simulink model "MPC_Validation_2"  (R2020a)
settings: Solver=FixedStepAuto  StartTime=0.0  StopTime=tsim  FixedStep=baseRate  RelTol=1e-3  EnableMultiTasking=on
values from neighbouring files (symbols this model uses):
  Ad = -C(7:12,4:9)    [theFastMPCSolver3.m]
  ALGORITHM = 5    [Run_Initializer.m]    (also in main.m = 7)
  baseRate = 0.05    [Run_Initializer.m]
  con0 = [n*N, 2*N, N, N, N]    [Run_Initializer.m]    (also in main.m)
  drop_states_ARM = [ pi/2, pi/2, 0]    [Run_Initializer.m]
  drop_states_BLACK = rand([1,3])/10+init_states_BLACK    [Run_Initializer.m]
  drop_states_BLUE = rand([1,3])/10+init_states_BLUE    [Run_Initializer.m]
  drop_states_RED = rand([1,3])/10+init_states_RED    [Run_Initializer.m]
  F_Black_X_nominal = 0.2196    [Run_Initializer.m]
  F_Black_Y_nominal = 0.2825    [Run_Initializer.m]
  F_Blue_X_nominal = 0.2196    [Run_Initializer.m]
  F_Blue_Y_nominal = 0.2825    [Run_Initializer.m]
  F_red_X_nominal = 0.2196    [Run_Initializer.m]
  F_red_Y_nominal = 0.2825    [Run_Initializer.m]
  F_thrusters_BLACK = [F_Black_X_nominal; F_Black_X_nominal;                             F_Black_Y_nominal; F_Black_Y_nominal; F_Black_X_nominal;                              F_Black_X_nominal; F_Black_Y_nominal; F_Black_Y_nominal]    [Run_Initializer.m]
  F_thrusters_BLUE = [F_Blue_X_nominal; F_Blue_X_nominal;                             F_Blue_Y_nominal; F_Blue_Y_nominal; F_Blue_X_nominal;                              F_Blue_X_nominal; F_Blue_Y_nominal; F_Blue_Y_nominal]    [Run_Initializer.m]
  F_thrusters_RED = [F_red_X_nominal; F_red_X_nominal;                             F_red_Y_nominal; F_red_Y_nominal; F_red_X_nominal;                              F_red_X_nominal; F_red_Y_nominal; F_red_Y_nominal]    [Run_Initializer.m]
  gamma = r - (excess + shrink + bracketwidth)    [theChaserSpacecraft.m]    (also in theTargetSpacecraft.m)
  Gamma1 = 0.0025    [Run_Initializer.m]
  Gamma2 = 100    [Run_Initializer.m]
  Gamma3 = 10    [Run_Initializer.m]
  Gamma4 = 0.001    [Run_Initializer.m]
  Gamma5 = 100    [Run_Initializer.m]
  Gamma6 = 0.001    [Run_Initializer.m]
  init_states_BLACK = [ct;thetat0].'    [Run_Initializer.m]
  init_states_BLUE = [pobj1;0].'    [Run_Initializer.m]
  init_states_RED = xi(1:3).'    [Run_Initializer.m]
  Kd_elarm = 0.05    [Run_Initializer.m]
  Kd_sharm = 0.05    [Run_Initializer.m]
  Kd_tb = 0.4    [Run_Initializer.m]
  Kd_tblue = 0.4    [Run_Initializer.m]
  Kd_tr = 0.4    [Run_Initializer.m]
  Kd_wrarm = 0.005    [Run_Initializer.m]
  Kd_xb = 8    [Run_Initializer.m]
  Kd_xblue = 8    [Run_Initializer.m]
  Kd_xr = 8    [Run_Initializer.m]
  Kd_yb = 8    [Run_Initializer.m]
  Kd_yblue = 8    [Run_Initializer.m]
  Kd_yr = 8    [Run_Initializer.m]
  Kp = [0.08 0 0 ... (first row only)    [Run_Initializer.m]
  Kp_elarm = 0.08    [Run_Initializer.m]
  Kp_sharm = 0.15    [Run_Initializer.m]
  Kp_tb = 0.1    [Run_Initializer.m]
  Kp_tblue = 0.1    [Run_Initializer.m]
  Kp_tr = 0.1    [Run_Initializer.m]
  Kp_wrarm = 0.007    [Run_Initializer.m]
  Kp_xb = 2    [Run_Initializer.m]
  Kp_xblue = 2    [Run_Initializer.m]
  Kp_xr = 2    [Run_Initializer.m]
  Kp_yb = 2    [Run_Initializer.m]
  Kp_yblue = 2    [Run_Initializer.m]
  Kp_yr = 2    [Run_Initializer.m]
  Kv = [0.05 0 0 ... (first row only)    [Run_Initializer.m]
  maxiterations = 10    [Run_Initializer.m]    (also in main.m)
  N = 15    [Run_Initializer.m]    (also in main.m; theFastMPCSolver2.m = length(z)/9; theFastMPCSolver3.m = length(z)/9)
  n = size(b,1)    [theFastMPCSolver3.m]
  noise_variance_BLACK = 0    [Run_Initializer.m]
  noise_variance_BLUE = 0    [Run_Initializer.m]
  noise_variance_RED = 0    [Run_Initializer.m]
  Phase0_End = Phase0_Duration    (= 5)    [Run_Initializer.m]
  Phase1_End = Phase0_Duration + Phase1_Duration    (= 10)    [Run_Initializer.m]
  Phase2_End = Phase0_Duration + Phase1_Duration +                                   Phase2_Duration    (= 36)    [Run_Initializer.m]
  Phase3_End = Phase0_Duration + Phase1_Duration +                                   Phase2_Duration + Phase3_Duration    (= 166)    [Run_Initializer.m]
  Phase3_SubPhase1_End = Phase2_End + Phase3_SubPhase1_Duration    (= 40)    [Run_Initializer.m]
  Phase3_SubPhase2_End = Phase2_End + Phase3_SubPhase1_Duration +                                   Phase3_SubPhase2_Duration    (= 42)    [Run_Initializer.m]
  Phase3_SubPhase3_End = Phase2_End + Phase3_SubPhase1_Duration +                                   Phase3_SubPhase2_Duration +                                  Phase3_SubPhase3_Duration    (= 44)    [Run_Initializer.m]
  Phase3_SubPhase4_End = Phase2_End + Phase3_SubPhase1_Duration +                                   Phase3_SubPhase2_Duration +                                  Phase3_SubPhase3_Duration +                                  Phase3_SubPhase4_Duration    [Run_Initializer.m]
  Phase4_End = Phase0_Duration + Phase1_Duration +                                   Phase2_Duration + Phase3_Duration +                                   Phase4_Duration    (= 186)    [Run_Initializer.m]
  Phase5_End = Phase0_Duration + Phase1_Duration +                                   Phase2_Duration + Phase3_Duration +                                   Phase4_Duration + Phase5_Duration    (= 191)    [Run_Initializer.m]
  serverRate = 0.1    [Run_Initializer.m]
  Td = 2    [Run_Initializer.m]    (also in main.m)
  thetat_dot = 0 * d2r    (= 0)    [Run_Initializer.m]    (also in main.m = -2.0 * d2r)
  thruster_dist2CG_BLACK = [83.42;-52.58;55.94;-60.05;54.08;-53.92;77.06;-55.94]    [Run_Initializer.m]
  thruster_dist2CG_BLUE = [73.54;-64.46;81.39;-60.11;64.46;-65.94;54.61;-74.39]    [Run_Initializer.m]
  thruster_dist2CG_RED = [49.92;-78.08;70.46;-63.54;81.08;-50.42;57.44;-75.96]    [Run_Initializer.m]
  tol = 0.00015    [Run_Initializer.m]    (also in main.m)
  Tz_lim_elarm = .1    (= 0.1)    [Run_Initializer.m]
  Tz_lim_sharm = .1    (= 0.1)    [Run_Initializer.m]
  Tz_lim_wrarm = .1    (= 0.1)    [Run_Initializer.m]
  vobj1 = [0.00;0.00]    [Run_Initializer.m]    (also in main.m)
  vtar = [0.0;0.0]    [Run_Initializer.m]    (also in main.m = [-0.008;0.008])
undefined symbols (not defined in the file or in its folder): cdockdeltax, cdockoa, Cmat, DiscIntNeverNeededParam, ecoa, Fmat, H, KOZ_actual, model_param, pdockoa, pdockr, platformSelection, rcone, rdock, simMode, Sj, taumax, thetah, Umat, umax, WhoAmI
libraries: dspstat3 x23, dspsigops x15, embdlinuxlib x10, raspberrypiBasiclib x10, simulink x8, MainLibrary x7, mspfiltlib x3, dsparch4 x3, dspswit3 x2, sensehatlib x1
(part 7 of 14)

== system MPC_Validation_2/IMU Data and Algorithms/Change RED Behavior/Fix Initial Bias/Correct GyroZ ==
  In1 : Inport
  Calculate Running Mean : Subsystem  TreatAsAtomicUnit=on
  Compare To Zero1 : simulink/Logic and Bit Operations/Compare To Zero  relop===  OutDataTypeStr=boolean
  Data Store Read1 : DataStoreRead  DataStoreName=RED_Rz
  Data Store Read3 : DataStoreRead  DataStoreName=RED_IMU_R
  Discrete-Time Integrator1 : DiscreteIntegrator  IntegratorMethod=Integration: Backward Euler  ExternalReset=either  InitialConditionSource=external  SampleTime=-1  ICPrevOutput=DiscIntNeverNeededParam  ICPrevScaledInput=DiscIntNeverNeededParam
  If : If  IfExpression=u1 < 5
  Pass Current Gyro : Subsystem  TreatAsAtomicUnit=on
  RED_Px4 : DataStoreWrite  DataStoreName=RED_IMU_Psi
  Subsystem : Subsystem
  Subtract : Sum  Inputs=+-
  Out1 : Outport
  wires:
  Subtract/1 -> Out1/1
  Subsystem/1(Time) -> If/1
  If/2 -> Pass Current Gyro/Action
  In1/1 -> Calculate Running Mean/1(In1), Pass Current Gyro/1(In1)
  If/1 -> Calculate Running Mean/Action
  Calculate Running Mean/1(Out1) -> Subtract/2
  Discrete-Time Integrator1/1 -> RED_Px4/1
  Compare To Zero1/1 -> Discrete-Time Integrator1/2
  Pass Current Gyro/1(Out1) -> Compare To Zero1/1, Subtract/1
  Data Store Read3/1 -> Discrete-Time Integrator1/1
  Data Store Read1/1 -> Discrete-Time Integrator1/3

== system MPC_Validation_2/IMU Data and Algorithms/Change RED Behavior/Fix Initial Bias (Accel)/Correct AccelX ==
  In1 : Inport
  Calculate Running Mean : Subsystem  TreatAsAtomicUnit=on
  If : If  IfExpression=u1 < 5
  Pass Current Accel : Subsystem  TreatAsAtomicUnit=on
  Subsystem : Subsystem
  Subtract : Sum  Inputs=+-
  Out1 : Outport
  wires:
  Subtract/1 -> Out1/1
  Subsystem/1(Time) -> If/1
  If/2 -> Pass Current Accel/Action
  In1/1 -> Calculate Running Mean/1(In1), Pass Current Accel/1(In1)
  If/1 -> Calculate Running Mean/Action
  Pass Current Accel/1(Out1) -> Subtract/1
  Calculate Running Mean/1(Out1) -> Subtract/2

== system MPC_Validation_2/IMU Data and Algorithms/Change RED Behavior/Fix Initial Bias (Accel)/Correct AccelY ==
  In1 : Inport
  Calculate Running Mean : Subsystem  TreatAsAtomicUnit=on
  If : If  IfExpression=u1 < 5
  Pass Current Accel : Subsystem  TreatAsAtomicUnit=on
  Subsystem : Subsystem
  Subtract : Sum  Inputs=+-
  Out1 : Outport
  wires:
  Subtract/1 -> Out1/1
  Subsystem/1(Time) -> If/1
  If/2 -> Pass Current Accel/Action
  In1/1 -> Calculate Running Mean/1(In1), Pass Current Accel/1(In1)
  If/1 -> Calculate Running Mean/Action
  Pass Current Accel/1(Out1) -> Subtract/1
  Calculate Running Mean/1(Out1) -> Subtract/2

== system MPC_Validation_2/IMU Data and Algorithms/Change RED Behavior/Fix Initial Bias (Accel)/Correct AccelZ ==
  In1 : Inport
  Calculate Running Mean : Subsystem  TreatAsAtomicUnit=on
  If : If  IfExpression=u1 < 5
  Pass Current Accel : Subsystem  TreatAsAtomicUnit=on
  Subsystem : Subsystem
  Subtract : Sum  Inputs=+-
  Out1 : Outport
  wires:
  Subtract/1 -> Out1/1
  Subsystem/1(Time) -> If/1
  If/2 -> Pass Current Accel/Action
  In1/1 -> Calculate Running Mean/1(In1), Pass Current Accel/1(In1)
  If/1 -> Calculate Running Mean/Action
  Pass Current Accel/1(Out1) -> Subtract/1
  Calculate Running Mean/1(Out1) -> Subtract/2

== system MPC_Validation_2/Phase #2: Move to Initial Position/Change BLACK Behavior/Custom Discrete PD (Attitude)/x_dot -> x1 ==
  note: dy/dt ~= (y2-y1)/deltaT
  y(t) : Inport
  Delay1 : Delay  DelayLength=1  InitialConditionSource=Input port
      settings: InputPortMap=u0,p4
  Hold this value : Subsystem  TreatAsAtomicUnit=on
  Sum6 : Sum  Inputs=-+|
  divide by delta T : Gain  Gain=1/serverRate
  "if we went through a \"step\"" : If  IfExpression=u1 ~= 0  ShowElse=off
  dy(t)/dt : Outport  VectorParamsAs1DForOutWhenUnconnected=off
  wires:
  divide by delta T/1 -> dy(t)/dt/1
  Delay1/1 -> Sum6/1
  "if we went through a \"step\""/1 -> Hold this value/Action
  Hold this value/1(Out1) -> divide by delta T/1
  Sum6/1 -> "if we went through a \"step\""/1, Hold this value/1(In1)
  y(t)/1 -> Sum6/2, Delay1/2, Delay1/1

== system MPC_Validation_2/Phase #2: Move to Initial Position/Change BLACK Behavior/Custom Discrete PD (X-Position)/x_dot -> x1 ==
  note: dy/dt ~= (y2-y1)/deltaT
  y(t) : Inport
  Delay1 : Delay  DelayLength=1  InitialConditionSource=Input port
      settings: InputPortMap=u0,p4
  Hold this value : Subsystem  TreatAsAtomicUnit=on
  Sum6 : Sum  Inputs=-+|
  divide by delta T : Gain  Gain=1/serverRate
  "if we went through a \"step\"" : If  IfExpression=u1 ~= 0  ShowElse=off
  dy(t)/dt : Outport  VectorParamsAs1DForOutWhenUnconnected=off
  wires:
  divide by delta T/1 -> dy(t)/dt/1
  Delay1/1 -> Sum6/1
  "if we went through a \"step\""/1 -> Hold this value/Action
  Hold this value/1(Out1) -> divide by delta T/1
  Sum6/1 -> "if we went through a \"step\""/1, Hold this value/1(In1)
  y(t)/1 -> Sum6/2, Delay1/2, Delay1/1

== system MPC_Validation_2/Phase #2: Move to Initial Position/Change BLACK Behavior/Custom Discrete PD (Y-Position)/x_dot -> x1 ==
  note: dy/dt ~= (y2-y1)/deltaT
  y(t) : Inport
  Delay1 : Delay  DelayLength=1  InitialConditionSource=Input port
      settings: InputPortMap=u0,p4
  Hold this value : Subsystem  TreatAsAtomicUnit=on
  Sum6 : Sum  Inputs=-+|
  divide by delta T : Gain  Gain=1/serverRate
  "if we went through a \"step\"" : If  IfExpression=u1 ~= 0  ShowElse=off
  dy(t)/dt : Outport  VectorParamsAs1DForOutWhenUnconnected=off
  wires:
  divide by delta T/1 -> dy(t)/dt/1
  Delay1/1 -> Sum6/1
  "if we went through a \"step\""/1 -> Hold this value/Action
  Hold this value/1(Out1) -> divide by delta T/1
  Sum6/1 -> "if we went through a \"step\""/1, Hold this value/1(In1)
  y(t)/1 -> Sum6/2, Delay1/2, Delay1/1

== system MPC_Validation_2/Phase #2: Move to Initial Position/Change BLUE Behavior/Custom Discrete PD (Attitude)/x_dot -> x1 ==
  note: dy/dt ~= (y2-y1)/deltaT
  y(t) : Inport
  Delay1 : Delay  DelayLength=1  InitialConditionSource=Input port
      settings: InputPortMap=u0,p4
  Hold this value : Subsystem  TreatAsAtomicUnit=on
  Sum6 : Sum  Inputs=-+|
  divide by delta T : Gain  Gain=1/serverRate
  "if we went through a \"step\"" : If  IfExpression=u1 ~= 0  ShowElse=off
  dy(t)/dt : Outport  VectorParamsAs1DForOutWhenUnconnected=off
  wires:
  divide by delta T/1 -> dy(t)/dt/1
  Delay1/1 -> Sum6/1
  "if we went through a \"step\""/1 -> Hold this value/Action
  Hold this value/1(Out1) -> divide by delta T/1
  Sum6/1 -> "if we went through a \"step\""/1, Hold this value/1(In1)
  y(t)/1 -> Sum6/2, Delay1/2, Delay1/1

== system MPC_Validation_2/Phase #2: Move to Initial Position/Change BLUE Behavior/Custom Discrete PD (X-Position)/x_dot -> x1 ==
  note: dy/dt ~= (y2-y1)/deltaT
  y(t) : Inport
  Delay1 : Delay  DelayLength=1  InitialConditionSource=Input port
      settings: InputPortMap=u0,p4
  Hold this value : Subsystem  TreatAsAtomicUnit=on
  Sum6 : Sum  Inputs=-+|
  divide by delta T : Gain  Gain=1/serverRate
  "if we went through a \"step\"" : If  IfExpression=u1 ~= 0  ShowElse=off
  dy(t)/dt : Outport  VectorParamsAs1DForOutWhenUnconnected=off
  wires:
  divide by delta T/1 -> dy(t)/dt/1
  Delay1/1 -> Sum6/1
  "if we went through a \"step\""/1 -> Hold this value/Action
  Hold this value/1(Out1) -> divide by delta T/1
  Sum6/1 -> "if we went through a \"step\""/1, Hold this value/1(In1)
  y(t)/1 -> Sum6/2, Delay1/2, Delay1/1

== system MPC_Validation_2/Phase #2: Move to Initial Position/Change BLUE Behavior/Custom Discrete PD (Y-Position)/x_dot -> x1 ==
  note: dy/dt ~= (y2-y1)/deltaT
  y(t) : Inport
  Delay1 : Delay  DelayLength=1  InitialConditionSource=Input port
      settings: InputPortMap=u0,p4
  Hold this value : Subsystem  TreatAsAtomicUnit=on
  Sum6 : Sum  Inputs=-+|
  divide by delta T : Gain  Gain=1/serverRate
  "if we went through a \"step\"" : If  IfExpression=u1 ~= 0  ShowElse=off
  dy(t)/dt : Outport  VectorParamsAs1DForOutWhenUnconnected=off
  wires:
  divide by delta T/1 -> dy(t)/dt/1
  Delay1/1 -> Sum6/1
  "if we went through a \"step\""/1 -> Hold this value/Action
  Hold this value/1(Out1) -> divide by delta T/1
  Sum6/1 -> "if we went through a \"step\""/1, Hold this value/1(In1)
  y(t)/1 -> Sum6/2, Delay1/2, Delay1/1

== system MPC_Validation_2/Phase #2: Move to Initial Position/Change RED Behavior/Custom Discrete PD (Attitude)/x_dot -> x1 ==
  note: dy/dt ~= (y2-y1)/deltaT
  y(t) : Inport
  Delay1 : Delay  DelayLength=1  InitialConditionSource=Input port
      settings: InputPortMap=u0,p4
  Hold this value : Subsystem  TreatAsAtomicUnit=on
  Sum6 : Sum  Inputs=-+|
  divide by delta T : Gain  Gain=1/serverRate
  "if we went through a \"step\"" : If  IfExpression=u1 ~= 0  ShowElse=off
  dy(t)/dt : Outport  VectorParamsAs1DForOutWhenUnconnected=off
  wires:
  divide by delta T/1 -> dy(t)/dt/1
  Delay1/1 -> Sum6/1
  "if we went through a \"step\""/1 -> Hold this value/Action
  Hold this value/1(Out1) -> divide by delta T/1
  Sum6/1 -> "if we went through a \"step\""/1, Hold this value/1(In1)
  y(t)/1 -> Sum6/2, Delay1/2, Delay1/1

== system MPC_Validation_2/Phase #2: Move to Initial Position/Change RED Behavior/Custom Discrete PD (X-Position)/x_dot -> x1 ==
  note: dy/dt ~= (y2-y1)/deltaT
  y(t) : Inport
  Delay1 : Delay  DelayLength=1  InitialConditionSource=Input port
      settings: InputPortMap=u0,p4
  Hold this value : Subsystem  TreatAsAtomicUnit=on
  Sum6 : Sum  Inputs=-+|
  divide by delta T : Gain  Gain=1/serverRate
  "if we went through a \"step\"" : If  IfExpression=u1 ~= 0  ShowElse=off
  dy(t)/dt : Outport  VectorParamsAs1DForOutWhenUnconnected=off
  wires:
  divide by delta T/1 -> dy(t)/dt/1
  Delay1/1 -> Sum6/1
  "if we went through a \"step\""/1 -> Hold this value/Action
  Hold this value/1(Out1) -> divide by delta T/1
  Sum6/1 -> "if we went through a \"step\""/1, Hold this value/1(In1)
  y(t)/1 -> Sum6/2, Delay1/2, Delay1/1

== system MPC_Validation_2/Phase #2: Move to Initial Position/Change RED Behavior/Custom Discrete PD (Y-Position)/x_dot -> x1 ==
  note: dy/dt ~= (y2-y1)/deltaT
  y(t) : Inport
  Delay1 : Delay  DelayLength=1  InitialConditionSource=Input port
      settings: InputPortMap=u0,p4
  Hold this value : Subsystem  TreatAsAtomicUnit=on
  Sum6 : Sum  Inputs=-+|
  divide by delta T : Gain  Gain=1/serverRate
  "if we went through a \"step\"" : If  IfExpression=u1 ~= 0  ShowElse=off
  dy(t)/dt : Outport  VectorParamsAs1DForOutWhenUnconnected=off
  wires:
  divide by delta T/1 -> dy(t)/dt/1
  Delay1/1 -> Sum6/1
  "if we went through a \"step\""/1 -> Hold this value/Action
  Hold this value/1(Out1) -> divide by delta T/1
  Sum6/1 -> "if we went through a \"step\""/1, Hold this value/1(In1)
  y(t)/1 -> Sum6/2, Delay1/2, Delay1/1

== system MPC_Validation_2/Phase #2: Move to Initial Position/Change RED Behavior/RED+ARM/Custom Discrete PD (X-Position)1 ==
  ex : Inport
  Sum3 : Sum
  kd_xr : Gain  Gain=Kd_sharm
  kp_xr : Gain  Gain=Kp_sharm
  "x_dot -> x1" : Subsystem
  Fx : Outport  VectorParamsAs1DForOutWhenUnconnected=off
  wires:
  kd_xr/1 -> Sum3/1
  ex/1 -> "x_dot -> x1"/1(y(t)), kp_xr/1
  kp_xr/1 -> Sum3/2
  "x_dot -> x1"/1(dy(t)/dt) -> kd_xr/1
  Sum3/1 -> Fx/1

== system MPC_Validation_2/Phase #2: Move to Initial Position/Change RED Behavior/RED+ARM/Custom Discrete PD (Y-Position)1 ==
  ey : Inport
  Sum3 : Sum
  kd_yr : Gain  Gain=Kd_elarm
  kp_yr : Gain  Gain=Kp_elarm
  "x_dot -> x1" : Subsystem
  Fy : Outport  VectorParamsAs1DForOutWhenUnconnected=off
  wires:
  kd_yr/1 -> Sum3/1
  Sum3/1 -> Fy/1
  kp_yr/1 -> Sum3/2
  "x_dot -> x1"/1(dy(t)/dt) -> kd_yr/1
  ey/1 -> "x_dot -> x1"/1(y(t)), kp_yr/1

== system MPC_Validation_2/Phase #2: Move to Initial Position/Change RED Behavior/RED+ARM/Custom Discrete PD (Y-Position)2 ==
  ey : Inport
  Sum3 : Sum
  kd_yr : Gain  Gain=Kd_wrarm
  kp_yr : Gain  Gain=Kp_wrarm
  "x_dot -> x1" : Subsystem
  Fy : Outport  VectorParamsAs1DForOutWhenUnconnected=off
  wires:
  kd_yr/1 -> Sum3/1
  Sum3/1 -> Fy/1
  kp_yr/1 -> Sum3/2
  "x_dot -> x1"/1(dy(t)/dt) -> kd_yr/1
  ey/1 -> "x_dot -> x1"/1(y(t)), kp_yr/1

== system MPC_Validation_2/Phase #3: Experiment/Change BLACK Behavior/Sub-Phase #1/Custom Discrete PD (Attitude) ==
  ez : Inport
  Sum3 : Sum
  kd_tb : Gain  Gain=Kd_tb
  kp_tb : Gain  Gain=Kp_tb
  "x_dot -> x1" : Subsystem
  Tz : Outport  VectorParamsAs1DForOutWhenUnconnected=off
  wires:
  kd_tb/1 -> Sum3/1
  Sum3/1 -> Tz/1
  kp_tb/1 -> Sum3/2
  "x_dot -> x1"/1(dy(t)/dt) -> kd_tb/1
  ez/1 -> "x_dot -> x1"/1(y(t)), kp_tb/1

== system MPC_Validation_2/Phase #3: Experiment/Change BLACK Behavior/Sub-Phase #1/Custom Discrete PD (X-Position) ==
  ex : Inport
  Sum3 : Sum
  kd_xb : Gain  Gain=Kd_xb
  kp_xb : Gain  Gain=Kp_xb
  "x_dot -> x1" : Subsystem
  Fx : Outport  VectorParamsAs1DForOutWhenUnconnected=off
  wires:
  kd_xb/1 -> Sum3/1
  ex/1 -> "x_dot -> x1"/1(y(t)), kp_xb/1
  kp_xb/1 -> Sum3/2
  "x_dot -> x1"/1(dy(t)/dt) -> kd_xb/1
  Sum3/1 -> Fx/1

== system MPC_Validation_2/Phase #3: Experiment/Change BLACK Behavior/Sub-Phase #1/Custom Discrete PD (Y-Position) ==
  ey : Inport
  Sum3 : Sum
  kd_yb : Gain  Gain=Kd_yb
  kp_yb : Gain  Gain=Kp_yb
  "x_dot -> x1" : Subsystem
  Fy : Outport  VectorParamsAs1DForOutWhenUnconnected=off
  wires:
  kd_yb/1 -> Sum3/1
  Sum3/1 -> Fy/1
  kp_yb/1 -> Sum3/2
  "x_dot -> x1"/1(dy(t)/dt) -> kd_yb/1
  ey/1 -> "x_dot -> x1"/1(y(t)), kp_yb/1

== system MPC_Validation_2/Phase #3: Experiment/Change BLACK Behavior/Sub-Phase #1/Hough Control ==
  Ref : Inport
  Act : Inport  Port=2
  MATLAB Function2 : MATLAB Function  TreatAsAtomicUnit=on
  MATLAB Function3 : MATLAB Function  TreatAsAtomicUnit=on
  MATLAB Function4 : MATLAB Function  TreatAsAtomicUnit=on
  Subtract2 : Sum  Inputs=+-
  Err : Outport  VectorParamsAs1DForOutWhenUnconnected=off
  wires:
  MATLAB Function4/1(e_out) -> Err/1
  MATLAB Function2/1(Oy) -> MATLAB Function4/1(Oy)
  Subtract2/1 -> MATLAB Function4/2(e_in)
  MATLAB Function2/2(Ox) -> Subtract2/1
  Act/1 -> MATLAB Function3/1(z)
  Ref/1 -> MATLAB Function2/1(z)
  MATLAB Function3/1(Ox) -> Subtract2/2

== system MPC_Validation_2/Phase #3: Experiment/Change BLACK Behavior/Sub-Phase #2 /Custom Discrete PD (Attitude) ==
  ez : Inport
  Sum3 : Sum
  kd_tb : Gain  Gain=Kd_tb
  kp_tb : Gain  Gain=Kp_tb
  "x_dot -> x1" : Subsystem
  Tz : Outport  VectorParamsAs1DForOutWhenUnconnected=off
  wires:
  kd_tb/1 -> Sum3/1
  Sum3/1 -> Tz/1
  kp_tb/1 -> Sum3/2
  "x_dot -> x1"/1(dy(t)/dt) -> kd_tb/1
  ez/1 -> "x_dot -> x1"/1(y(t)), kp_tb/1

== system MPC_Validation_2/Phase #3: Experiment/Change BLACK Behavior/Sub-Phase #2 /Custom Discrete PD (X-Position) ==
  ex : Inport
  Sum3 : Sum
  kd_xb : Gain  Gain=Kd_xb
  kp_xb : Gain  Gain=Kp_xb
  "x_dot -> x1" : Subsystem
  Fx : Outport  VectorParamsAs1DForOutWhenUnconnected=off
  wires:
  kd_xb/1 -> Sum3/1
  ex/1 -> "x_dot -> x1"/1(y(t)), kp_xb/1
  kp_xb/1 -> Sum3/2
  "x_dot -> x1"/1(dy(t)/dt) -> kd_xb/1
  Sum3/1 -> Fx/1

== system MPC_Validation_2/Phase #3: Experiment/Change BLACK Behavior/Sub-Phase #2 /Custom Discrete PD (Y-Position) ==
  ey : Inport
  Sum3 : Sum
  kd_yb : Gain  Gain=Kd_yb
  kp_yb : Gain  Gain=Kp_yb
  "x_dot -> x1" : Subsystem
  Fy : Outport  VectorParamsAs1DForOutWhenUnconnected=off
  wires:
  kd_yb/1 -> Sum3/1
  Sum3/1 -> Fy/1
  kp_yb/1 -> Sum3/2
  "x_dot -> x1"/1(dy(t)/dt) -> kd_yb/1
  ey/1 -> "x_dot -> x1"/1(y(t)), kp_yb/1

== system MPC_Validation_2/Phase #3: Experiment/Change BLACK Behavior/Sub-Phase #2 /Hough Control ==
  Ref : Inport
  Act : Inport  Port=2
  MATLAB Function2 : MATLAB Function  TreatAsAtomicUnit=on
  MATLAB Function3 : MATLAB Function  TreatAsAtomicUnit=on
  MATLAB Function4 : MATLAB Function  TreatAsAtomicUnit=on
  Subtract2 : Sum  Inputs=+-
  Err : Outport  VectorParamsAs1DForOutWhenUnconnected=off
  wires:
  MATLAB Function4/1(e_out) -> Err/1
  MATLAB Function2/1(Oy) -> MATLAB Function4/1(Oy)
  Subtract2/1 -> MATLAB Function4/2(e_in)
  MATLAB Function2/2(Ox) -> Subtract2/1
  Act/1 -> MATLAB Function3/1(z)
  Ref/1 -> MATLAB Function2/1(z)
  MATLAB Function3/1(Ox) -> Subtract2/2

== system MPC_Validation_2/Phase #3: Experiment/Change BLACK Behavior/Sub-Phase #3 /Custom Discrete PD (Attitude) ==
  ez : Inport
  Sum3 : Sum
  kd_tb : Gain  Gain=Kd_tb
  kp_tb : Gain  Gain=Kp_tb
  "x_dot -> x1" : Subsystem
  Tz : Outport  VectorParamsAs1DForOutWhenUnconnected=off
  wires:
  kd_tb/1 -> Sum3/1
  Sum3/1 -> Tz/1
  kp_tb/1 -> Sum3/2
  "x_dot -> x1"/1(dy(t)/dt) -> kd_tb/1
  ez/1 -> "x_dot -> x1"/1(y(t)), kp_tb/1

== system MPC_Validation_2/Phase #3: Experiment/Change BLACK Behavior/Sub-Phase #3 /Custom Discrete PD (X-Position) ==
  ex : Inport
  Sum3 : Sum
  kd_xb : Gain  Gain=Kd_xb
  kp_xb : Gain  Gain=Kp_xb
  "x_dot -> x1" : Subsystem
  Fx : Outport  VectorParamsAs1DForOutWhenUnconnected=off
  wires:
  kd_xb/1 -> Sum3/1
  ex/1 -> "x_dot -> x1"/1(y(t)), kp_xb/1
  kp_xb/1 -> Sum3/2
  "x_dot -> x1"/1(dy(t)/dt) -> kd_xb/1
  Sum3/1 -> Fx/1

== system MPC_Validation_2/Phase #3: Experiment/Change BLACK Behavior/Sub-Phase #3 /Custom Discrete PD (Y-Position) ==
  ey : Inport
  Sum3 : Sum
  kd_yb : Gain  Gain=Kd_yb
  kp_yb : Gain  Gain=Kp_yb
  "x_dot -> x1" : Subsystem
  Fy : Outport  VectorParamsAs1DForOutWhenUnconnected=off
  wires:
  kd_yb/1 -> Sum3/1
  Sum3/1 -> Fy/1
  kp_yb/1 -> Sum3/2
  "x_dot -> x1"/1(dy(t)/dt) -> kd_yb/1
  ey/1 -> "x_dot -> x1"/1(y(t)), kp_yb/1

== system MPC_Validation_2/Phase #3: Experiment/Change BLACK Behavior/Sub-Phase #3 /Desired angle with spin ==
  Constant : Constant  Value=thetat_dot
  Constant1 : Constant  Value=Phase3_SubPhase2_End
  Constant2 : Constant  Commented=on  Value=Phase1_End
  Desired Attitude (BLACK) : Constant  Value=init_states_BLACK(3)  SampleTime=-1
  Product : Product
  Sum : Sum  Inputs=+-
  Sum1 : Sum
  Universal_Time : DataStoreRead  DataStoreName=Univ_Time
  Ref : Outport
  wires:
  Constant/1 -> Product/1
  Product/1 -> Sum1/2
  Constant1/1 -> Sum/2
  Sum/1 -> Product/2
  Universal_Time/1 -> Sum/1
  Sum1/1 -> Ref/1
  Desired Attitude (BLACK)/1 -> Sum1/1

== system MPC_Validation_2/Phase #3: Experiment/Change BLACK Behavior/Sub-Phase #3 /Desired x-pos ==
  Constant : Constant  Value=vtar
  Constant1 : Constant  Value=Phase3_SubPhase2_End
  Constant2 : Constant  Commented=on  Value=Phase1_End
  Demux : Demux  Outputs=2
  Desired Attitude (BLACK) : Constant  Value=init_states_BLACK(1)  SampleTime=-1
  Product : Product
  Sum : Sum  Inputs=+-
  Sum1 : Sum
  Terminator : Terminator
  Universal_Time : DataStoreRead  DataStoreName=Univ_Time
  Ref : Outport
  wires:
  Product/1 -> Sum1/2
  Constant1/1 -> Sum/2
  Sum/1 -> Product/2
  Universal_Time/1 -> Sum/1
  Sum1/1 -> Ref/1
  Desired Attitude (BLACK)/1 -> Sum1/1
  Constant/1 -> Demux/1
  Demux/1 -> Product/1
  Demux/2 -> Terminator/1

== system MPC_Validation_2/Phase #3: Experiment/Change BLACK Behavior/Sub-Phase #3 /Desired y-pos ==
  Constant : Constant  Value=vtar
  Constant1 : Constant  Value=Phase3_SubPhase2_End
  Constant2 : Constant  Commented=on  Value=Phase1_End
  Demux : Demux  Outputs=2
  Desired Attitude (BLACK) : Constant  Value=init_states_BLACK(2)  SampleTime=-1
  Product : Product
  Sum : Sum  Inputs=+-
  Sum1 : Sum
  Terminator : Terminator
  Universal_Time : DataStoreRead  DataStoreName=Univ_Time
  Ref : Outport
  wires:
  Product/1 -> Sum1/2
  Constant1/1 -> Sum/2
  Sum/1 -> Product/2
  Universal_Time/1 -> Sum/1
  Sum1/1 -> Ref/1
  Desired Attitude (BLACK)/1 -> Sum1/1
  Constant/1 -> Demux/1
  Demux/1 -> Terminator/1
  Demux/2 -> Product/1

== system MPC_Validation_2/Phase #3: Experiment/Change BLACK Behavior/Sub-Phase #3 /Hough Control ==
  Ref : Inport
  Act : Inport  Port=2
  MATLAB Function2 : MATLAB Function  TreatAsAtomicUnit=on
  MATLAB Function3 : MATLAB Function  TreatAsAtomicUnit=on
  MATLAB Function4 : MATLAB Function  TreatAsAtomicUnit=on
  Subtract2 : Sum  Inputs=+-
  Err : Outport  VectorParamsAs1DForOutWhenUnconnected=off
  wires:
  MATLAB Function4/1(e_out) -> Err/1
  MATLAB Function2/1(Oy) -> MATLAB Function4/1(Oy)
  Subtract2/1 -> MATLAB Function4/2(e_in)
  MATLAB Function2/2(Ox) -> Subtract2/1
  Act/1 -> MATLAB Function3/1(z)
  Ref/1 -> MATLAB Function2/1(z)
  MATLAB Function3/1(Ox) -> Subtract2/2

== system MPC_Validation_2/Phase #3: Experiment/Change BLACK Behavior/Sub-Phase #4/BLACK_RzD ==
  Desired Rate (BLACK) : Constant  Value=0.104719755/2  SampleTime=-1
  Product : Product
  Subsystem : Subsystem
  Wrap1 : Subsystem
  Out1 : Outport  VectorParamsAs1DForOutWhenUnconnected=off
  wires:
  Wrap1/1(wrapped) -> Out1/1
  Desired Rate (BLACK)/1 -> Product/1
  Subsystem/1(Time) -> Product/2
  Product/1 -> Wrap1/1(unwrapped)

== system MPC_Validation_2/Phase #3: Experiment/Change BLACK Behavior/Sub-Phase #4/Custom Discrete PD (Attitude) ==
  ez : Inport
  Sum3 : Sum
  kd_tb : Gain  Gain=Kd_tb
  kp_tb : Gain  Gain=Kp_tb
  "x_dot -> x1" : Subsystem
  Tz : Outport  VectorParamsAs1DForOutWhenUnconnected=off
  wires:
  kd_tb/1 -> Sum3/1
  Sum3/1 -> Tz/1
  kp_tb/1 -> Sum3/2
  "x_dot -> x1"/1(dy(t)/dt) -> kd_tb/1
  ez/1 -> "x_dot -> x1"/1(y(t)), kp_tb/1

== system MPC_Validation_2/Phase #3: Experiment/Change BLACK Behavior/Sub-Phase #4/Custom Discrete PD (X-Position) ==
  ex : Inport
  Sum3 : Sum
  kd_xb : Gain  Gain=Kd_xb
  kp_xb : Gain  Gain=Kp_xb
  "x_dot -> x1" : Subsystem
  Fx : Outport  VectorParamsAs1DForOutWhenUnconnected=off
  wires:
  kd_xb/1 -> Sum3/1
  ex/1 -> "x_dot -> x1"/1(y(t)), kp_xb/1
  kp_xb/1 -> Sum3/2
  "x_dot -> x1"/1(dy(t)/dt) -> kd_xb/1
  Sum3/1 -> Fx/1

== system MPC_Validation_2/Phase #3: Experiment/Change BLACK Behavior/Sub-Phase #4/Custom Discrete PD (Y-Position) ==
  ey : Inport
  Sum3 : Sum
  kd_yb : Gain  Gain=Kd_yb
  kp_yb : Gain  Gain=Kp_yb
  "x_dot -> x1" : Subsystem
  Fy : Outport  VectorParamsAs1DForOutWhenUnconnected=off
  wires:
  kd_yb/1 -> Sum3/1
  Sum3/1 -> Fy/1
  kp_yb/1 -> Sum3/2
  "x_dot -> x1"/1(dy(t)/dt) -> kd_yb/1
  ey/1 -> "x_dot -> x1"/1(y(t)), kp_yb/1

== system MPC_Validation_2/Phase #3: Experiment/Change BLACK Behavior/Sub-Phase #4/Desired angle with spin ==
  Constant : Constant  Value=thetat_dot
  Constant1 : Constant  Value=Phase3_SubPhase2_End
  Constant2 : Constant  Commented=on  Value=Phase1_End
  Desired Attitude (BLACK) : Constant  Value=init_states_BLACK(3)  SampleTime=-1
  Product : Product
  Sum : Sum  Inputs=+-
  Sum1 : Sum
  Universal_Time : DataStoreRead  DataStoreName=Univ_Time
  Ref : Outport
  wires:
  Constant/1 -> Product/1
  Product/1 -> Sum1/2
  Constant1/1 -> Sum/2
  Sum/1 -> Product/2
  Universal_Time/1 -> Sum/1
  Sum1/1 -> Ref/1
  Desired Attitude (BLACK)/1 -> Sum1/1

== system MPC_Validation_2/Phase #3: Experiment/Change BLACK Behavior/Sub-Phase #4/Desired x-pos ==
  Constant : Constant  Value=vtar
  Constant1 : Constant  Value=Phase3_SubPhase2_End
  Constant2 : Constant  Commented=on  Value=Phase1_End
  Demux : Demux  Outputs=2
  Desired Attitude (BLACK) : Constant  Value=init_states_BLACK(1)  SampleTime=-1
  Product : Product
  Sum : Sum  Inputs=+-
  Sum1 : Sum
  Terminator : Terminator
  Universal_Time : DataStoreRead  DataStoreName=Univ_Time
  Ref : Outport
  wires:
  Product/1 -> Sum1/2
  Constant1/1 -> Sum/2
  Sum/1 -> Product/2
  Universal_Time/1 -> Sum/1
  Sum1/1 -> Ref/1
  Desired Attitude (BLACK)/1 -> Sum1/1
  Constant/1 -> Demux/1
  Demux/1 -> Product/1
  Demux/2 -> Terminator/1

== system MPC_Validation_2/Phase #3: Experiment/Change BLACK Behavior/Sub-Phase #4/Desired y-pos ==
  Constant : Constant  Value=vtar
  Constant1 : Constant  Value=Phase3_SubPhase2_End
  Constant2 : Constant  Commented=on  Value=Phase1_End
  Demux : Demux  Outputs=2
  Desired Attitude (BLACK) : Constant  Value=init_states_BLACK(2)  SampleTime=-1
  Product : Product
  Sum : Sum  Inputs=+-
  Sum1 : Sum
  Terminator : Terminator
  Universal_Time : DataStoreRead  DataStoreName=Univ_Time
  Ref : Outport
  wires:
  Product/1 -> Sum1/2
  Constant1/1 -> Sum/2
  Sum/1 -> Product/2
  Universal_Time/1 -> Sum/1
  Sum1/1 -> Ref/1
  Desired Attitude (BLACK)/1 -> Sum1/1
  Constant/1 -> Demux/1
  Demux/1 -> Terminator/1
  Demux/2 -> Product/1

== system MPC_Validation_2/Phase #3: Experiment/Change BLACK Behavior/Sub-Phase #4/Hough Control ==
  Ref : Inport
  Act : Inport  Port=2
  MATLAB Function2 : MATLAB Function  TreatAsAtomicUnit=on
  MATLAB Function3 : MATLAB Function  TreatAsAtomicUnit=on
  MATLAB Function4 : MATLAB Function  TreatAsAtomicUnit=on
  Subtract2 : Sum  Inputs=+-
  Err : Outport  VectorParamsAs1DForOutWhenUnconnected=off
  wires:
  MATLAB Function4/1(e_out) -> Err/1
  MATLAB Function2/1(Oy) -> MATLAB Function4/1(Oy)
  Subtract2/1 -> MATLAB Function4/2(e_in)
  MATLAB Function2/2(Ox) -> Subtract2/1
  Act/1 -> MATLAB Function3/1(z)
  Ref/1 -> MATLAB Function2/1(z)
  MATLAB Function3/1(Ox) -> Subtract2/2

== system MPC_Validation_2/Phase #3: Experiment/Change BLUE Behavior/Sub-Phase #1/Custom Discrete PD (Attitude) ==
  ez : Inport
  Sum3 : Sum
  kd_tb : Gain  Gain=Kd_tblue
  kp_tb : Gain  Gain=Kp_tblue
  "x_dot -> x1" : Subsystem
  Tz : Outport  VectorParamsAs1DForOutWhenUnconnected=off
  wires:
  kd_tb/1 -> Sum3/1
  Sum3/1 -> Tz/1
  kp_tb/1 -> Sum3/2
  "x_dot -> x1"/1(dy(t)/dt) -> kd_tb/1
  ez/1 -> "x_dot -> x1"/1(y(t)), kp_tb/1

== system MPC_Validation_2/Phase #3: Experiment/Change BLUE Behavior/Sub-Phase #1/Custom Discrete PD (X-Position) ==
  ex : Inport
  Sum3 : Sum
  kd_xb : Gain  Gain=Kd_xblue
  kp_xb : Gain  Gain=Kp_xblue
  "x_dot -> x1" : Subsystem
  Fx : Outport  VectorParamsAs1DForOutWhenUnconnected=off
  wires:
  kd_xb/1 -> Sum3/1
  ex/1 -> "x_dot -> x1"/1(y(t)), kp_xb/1
  kp_xb/1 -> Sum3/2
  "x_dot -> x1"/1(dy(t)/dt) -> kd_xb/1
  Sum3/1 -> Fx/1

== system MPC_Validation_2/Phase #3: Experiment/Change BLUE Behavior/Sub-Phase #1/Custom Discrete PD (Y-Position) ==
  ey : Inport
  Sum3 : Sum
  kd_yb : Gain  Gain=Kd_yblue
  kp_yb : Gain  Gain=Kp_yblue
  "x_dot -> x1" : Subsystem
  Fy : Outport  VectorParamsAs1DForOutWhenUnconnected=off
  wires:
  kd_yb/1 -> Sum3/1
  Sum3/1 -> Fy/1
  kp_yb/1 -> Sum3/2
  "x_dot -> x1"/1(dy(t)/dt) -> kd_yb/1
  ey/1 -> "x_dot -> x1"/1(y(t)), kp_yb/1

== system MPC_Validation_2/Phase #3: Experiment/Change BLUE Behavior/Sub-Phase #1/Hough Control ==
  Ref : Inport
  Act : Inport  Port=2
  MATLAB Function2 : MATLAB Function  TreatAsAtomicUnit=on
  MATLAB Function3 : MATLAB Function  TreatAsAtomicUnit=on
  MATLAB Function4 : MATLAB Function  TreatAsAtomicUnit=on
  Subtract2 : Sum  Inputs=+-
  Err : Outport  VectorParamsAs1DForOutWhenUnconnected=off
  wires:
  MATLAB Function4/1(e_out) -> Err/1
  MATLAB Function2/1(Oy) -> MATLAB Function4/1(Oy)
  Subtract2/1 -> MATLAB Function4/2(e_in)
  MATLAB Function2/2(Ox) -> Subtract2/1
  Act/1 -> MATLAB Function3/1(z)
  Ref/1 -> MATLAB Function2/1(z)
  MATLAB Function3/1(Ox) -> Subtract2/2

== system MPC_Validation_2/Phase #3: Experiment/Change BLUE Behavior/Sub-Phase #2 /Custom Discrete PD (Attitude) ==
  ez : Inport
  Sum3 : Sum
  kd_tb : Gain  Gain=Kd_tblue
  kp_tb : Gain  Gain=Kp_tblue
  "x_dot -> x1" : Subsystem
  Tz : Outport  VectorParamsAs1DForOutWhenUnconnected=off
  wires:
  kd_tb/1 -> Sum3/1
  Sum3/1 -> Tz/1
  kp_tb/1 -> Sum3/2
  "x_dot -> x1"/1(dy(t)/dt) -> kd_tb/1
  ez/1 -> "x_dot -> x1"/1(y(t)), kp_tb/1

== system MPC_Validation_2/Phase #3: Experiment/Change BLUE Behavior/Sub-Phase #2 /Custom Discrete PD (X-Position) ==
  ex : Inport
  Sum3 : Sum
  kd_xb : Gain  Gain=Kd_xblue
  kp_xb : Gain  Gain=Kp_xblue
  "x_dot -> x1" : Subsystem
  Fx : Outport  VectorParamsAs1DForOutWhenUnconnected=off
  wires:
  kd_xb/1 -> Sum3/1
  ex/1 -> "x_dot -> x1"/1(y(t)), kp_xb/1
  kp_xb/1 -> Sum3/2
  "x_dot -> x1"/1(dy(t)/dt) -> kd_xb/1
  Sum3/1 -> Fx/1

== system MPC_Validation_2/Phase #3: Experiment/Change BLUE Behavior/Sub-Phase #2 /Custom Discrete PD (Y-Position) ==
  ey : Inport
  Sum3 : Sum
  kd_yb : Gain  Gain=Kd_yblue
  kp_yb : Gain  Gain=Kp_yblue
  "x_dot -> x1" : Subsystem
  Fy : Outport  VectorParamsAs1DForOutWhenUnconnected=off
  wires:
  kd_yb/1 -> Sum3/1
  Sum3/1 -> Fy/1
  kp_yb/1 -> Sum3/2
  "x_dot -> x1"/1(dy(t)/dt) -> kd_yb/1
  ey/1 -> "x_dot -> x1"/1(y(t)), kp_yb/1

== system MPC_Validation_2/Phase #3: Experiment/Change BLUE Behavior/Sub-Phase #2 /Hough Control ==
  Ref : Inport
  Act : Inport  Port=2
  MATLAB Function2 : MATLAB Function  TreatAsAtomicUnit=on
  MATLAB Function3 : MATLAB Function  TreatAsAtomicUnit=on
  MATLAB Function4 : MATLAB Function  TreatAsAtomicUnit=on
  Subtract2 : Sum  Inputs=+-
  Err : Outport  VectorParamsAs1DForOutWhenUnconnected=off
  wires:
  MATLAB Function4/1(e_out) -> Err/1
  MATLAB Function2/1(Oy) -> MATLAB Function4/1(Oy)
  Subtract2/1 -> MATLAB Function4/2(e_in)
  MATLAB Function2/2(Ox) -> Subtract2/1
  Act/1 -> MATLAB Function3/1(z)
  Ref/1 -> MATLAB Function2/1(z)
  MATLAB Function3/1(Ox) -> Subtract2/2

== system MPC_Validation_2/Phase #3: Experiment/Change BLUE Behavior/Sub-Phase #3 /Custom Discrete PD (Attitude) ==
  ez : Inport
  Sum3 : Sum
  kd_tb : Gain  Gain=Kd_tblue
  kp_tb : Gain  Gain=Kp_tblue
  "x_dot -> x1" : Subsystem
  Tz : Outport  VectorParamsAs1DForOutWhenUnconnected=off
  wires:
  kd_tb/1 -> Sum3/1
  Sum3/1 -> Tz/1
  kp_tb/1 -> Sum3/2
  "x_dot -> x1"/1(dy(t)/dt) -> kd_tb/1
  ez/1 -> "x_dot -> x1"/1(y(t)), kp_tb/1

== system MPC_Validation_2/Phase #3: Experiment/Change BLUE Behavior/Sub-Phase #3 /Custom Discrete PD (X-Position) ==
  ex : Inport
  Sum3 : Sum
  kd_xb : Gain  Gain=Kd_xblue
  kp_xb : Gain  Gain=Kp_xblue
  "x_dot -> x1" : Subsystem
  Fx : Outport  VectorParamsAs1DForOutWhenUnconnected=off
  wires:
  kd_xb/1 -> Sum3/1
  ex/1 -> "x_dot -> x1"/1(y(t)), kp_xb/1
  kp_xb/1 -> Sum3/2
  "x_dot -> x1"/1(dy(t)/dt) -> kd_xb/1
  Sum3/1 -> Fx/1

== system MPC_Validation_2/Phase #3: Experiment/Change BLUE Behavior/Sub-Phase #3 /Custom Discrete PD (Y-Position) ==
  ey : Inport
  Sum3 : Sum
  kd_yb : Gain  Gain=Kd_yblue
  kp_yb : Gain  Gain=Kp_yblue
  "x_dot -> x1" : Subsystem
  Fy : Outport  VectorParamsAs1DForOutWhenUnconnected=off
  wires:
  kd_yb/1 -> Sum3/1
  Sum3/1 -> Fy/1
  kp_yb/1 -> Sum3/2
  "x_dot -> x1"/1(dy(t)/dt) -> kd_yb/1
  ey/1 -> "x_dot -> x1"/1(y(t)), kp_yb/1

== system MPC_Validation_2/Phase #3: Experiment/Change BLUE Behavior/Sub-Phase #3 /Desired x-pos ==
  Constant : Constant  Value=vobj1
  Constant1 : Constant  Value=Phase3_SubPhase2_End
  Constant2 : Constant  Commented=on  Value=Phase1_End
  Demux : Demux  Outputs=2
  Desired Attitude (BLACK) : Constant  Value=init_states_BLUE(1)  SampleTime=-1
  Product : Product
  Sum : Sum  Inputs=+-
  Sum1 : Sum
  Terminator : Terminator
  Universal_Time : DataStoreRead  DataStoreName=Univ_Time
  Ref : Outport
  wires:
  Product/1 -> Sum1/2
  Constant1/1 -> Sum/2
  Sum/1 -> Product/2
  Universal_Time/1 -> Sum/1
  Sum1/1 -> Ref/1
  Desired Attitude (BLACK)/1 -> Sum1/1
  Constant/1 -> Demux/1
  Demux/1 -> Product/1
  Demux/2 -> Terminator/1

== system MPC_Validation_2/Phase #3: Experiment/Change BLUE Behavior/Sub-Phase #3 /Desired y-pos ==
  Constant : Constant  Value=vobj1
  Constant1 : Constant  Value=Phase3_SubPhase2_End
  Constant2 : Constant  Commented=on  Value=Phase1_End
  Demux : Demux  Outputs=2
  Desired Attitude (BLACK) : Constant  Value=init_states_BLUE(2)  SampleTime=-1
  Product : Product
  Sum : Sum  Inputs=+-
  Sum1 : Sum
  Terminator : Terminator
  Universal_Time : DataStoreRead  DataStoreName=Univ_Time
  Ref : Outport
  wires:
  Product/1 -> Sum1/2
  Constant1/1 -> Sum/2
  Sum/1 -> Product/2
  Universal_Time/1 -> Sum/1
  Sum1/1 -> Ref/1
  Desired Attitude (BLACK)/1 -> Sum1/1
  Constant/1 -> Demux/1
  Demux/1 -> Terminator/1
  Demux/2 -> Product/1

== system MPC_Validation_2/Phase #3: Experiment/Change BLUE Behavior/Sub-Phase #3 /Hough Control ==
  Ref : Inport
  Act : Inport  Port=2
  MATLAB Function2 : MATLAB Function  TreatAsAtomicUnit=on
  MATLAB Function3 : MATLAB Function  TreatAsAtomicUnit=on
  MATLAB Function4 : MATLAB Function  TreatAsAtomicUnit=on
  Subtract2 : Sum  Inputs=+-
  Err : Outport  VectorParamsAs1DForOutWhenUnconnected=off
  wires:
  MATLAB Function4/1(e_out) -> Err/1
  MATLAB Function2/1(Oy) -> MATLAB Function4/1(Oy)
  Subtract2/1 -> MATLAB Function4/2(e_in)
  MATLAB Function2/2(Ox) -> Subtract2/1
  Act/1 -> MATLAB Function3/1(z)
  Ref/1 -> MATLAB Function2/1(z)
  MATLAB Function3/1(Ox) -> Subtract2/2

== system MPC_Validation_2/Phase #3: Experiment/Change BLUE Behavior/Sub-Phase #4/Custom Discrete PD (Attitude) ==
  ez : Inport
  Sum3 : Sum
  kd_tb : Gain  Gain=Kd_tblue
  kp_tb : Gain  Gain=Kp_tblue
  "x_dot -> x1" : Subsystem
  Tz : Outport  VectorParamsAs1DForOutWhenUnconnected=off
  wires:
  kd_tb/1 -> Sum3/1
  Sum3/1 -> Tz/1
  kp_tb/1 -> Sum3/2
  "x_dot -> x1"/1(dy(t)/dt) -> kd_tb/1
  ez/1 -> "x_dot -> x1"/1(y(t)), kp_tb/1

== system MPC_Validation_2/Phase #3: Experiment/Change BLUE Behavior/Sub-Phase #4/Custom Discrete PD (X-Position) ==
  ex : Inport
  Sum3 : Sum
  kd_xb : Gain  Gain=Kd_xblue
  kp_xb : Gain  Gain=Kp_xblue
  "x_dot -> x1" : Subsystem
  Fx : Outport  VectorParamsAs1DForOutWhenUnconnected=off
  wires:
  kd_xb/1 -> Sum3/1
  ex/1 -> "x_dot -> x1"/1(y(t)), kp_xb/1
  kp_xb/1 -> Sum3/2
  "x_dot -> x1"/1(dy(t)/dt) -> kd_xb/1
  Sum3/1 -> Fx/1

== system MPC_Validation_2/Phase #3: Experiment/Change BLUE Behavior/Sub-Phase #4/Custom Discrete PD (Y-Position) ==
  ey : Inport
  Sum3 : Sum
  kd_yb : Gain  Gain=Kd_yblue
  kp_yb : Gain  Gain=Kp_yblue
  "x_dot -> x1" : Subsystem
  Fy : Outport  VectorParamsAs1DForOutWhenUnconnected=off
  wires:
  kd_yb/1 -> Sum3/1
  Sum3/1 -> Fy/1
  kp_yb/1 -> Sum3/2
  "x_dot -> x1"/1(dy(t)/dt) -> kd_yb/1
  ey/1 -> "x_dot -> x1"/1(y(t)), kp_yb/1

== system MPC_Validation_2/Phase #3: Experiment/Change BLUE Behavior/Sub-Phase #4/Desired x-pos ==
  Constant : Constant  Value=vobj1
  Constant1 : Constant  Value=Phase3_SubPhase2_End
  Constant2 : Constant  Commented=on  Value=Phase1_End
  Demux : Demux  Outputs=2
  Desired Attitude (BLACK) : Constant  Value=init_states_BLUE(1)  SampleTime=-1
  Product : Product
  Sum : Sum  Inputs=+-
  Sum1 : Sum
  Terminator : Terminator
  Universal_Time : DataStoreRead  DataStoreName=Univ_Time
  Ref : Outport
  wires:
  Product/1 -> Sum1/2
  Constant1/1 -> Sum/2
  Sum/1 -> Product/2
  Universal_Time/1 -> Sum/1
  Sum1/1 -> Ref/1
  Desired Attitude (BLACK)/1 -> Sum1/1
  Constant/1 -> Demux/1
  Demux/1 -> Product/1
  Demux/2 -> Terminator/1

== system MPC_Validation_2/Phase #3: Experiment/Change BLUE Behavior/Sub-Phase #4/Desired y-pos ==
  Constant : Constant  Value=vobj1
  Constant1 : Constant  Value=Phase3_SubPhase2_End
  Constant2 : Constant  Commented=on  Value=Phase1_End
  Demux : Demux  Outputs=2
  Desired Attitude (BLACK) : Constant  Value=init_states_BLUE(2)  SampleTime=-1
  Product : Product
  Sum : Sum  Inputs=+-
  Sum1 : Sum
  Terminator : Terminator
  Universal_Time : DataStoreRead  DataStoreName=Univ_Time
  Ref : Outport
  wires:
  Product/1 -> Sum1/2
  Constant1/1 -> Sum/2
  Sum/1 -> Product/2
  Universal_Time/1 -> Sum/1
  Sum1/1 -> Ref/1
  Desired Attitude (BLACK)/1 -> Sum1/1
  Constant/1 -> Demux/1
  Demux/1 -> Terminator/1
  Demux/2 -> Product/1

== system MPC_Validation_2/Phase #3: Experiment/Change BLUE Behavior/Sub-Phase #4/Hough Control ==
  Ref : Inport
  Act : Inport  Port=2
  MATLAB Function2 : MATLAB Function  TreatAsAtomicUnit=on
  MATLAB Function3 : MATLAB Function  TreatAsAtomicUnit=on
  MATLAB Function4 : MATLAB Function  TreatAsAtomicUnit=on
  Subtract2 : Sum  Inputs=+-
  Err : Outport  VectorParamsAs1DForOutWhenUnconnected=off
  wires:
  MATLAB Function4/1(e_out) -> Err/1
  MATLAB Function2/1(Oy) -> MATLAB Function4/1(Oy)
  Subtract2/1 -> MATLAB Function4/2(e_in)
  MATLAB Function2/2(Ox) -> Subtract2/1
  Act/1 -> MATLAB Function3/1(z)
  Ref/1 -> MATLAB Function2/1(z)
  MATLAB Function3/1(Ox) -> Subtract2/2

== system MPC_Validation_2/Phase #3: Experiment/Change RED Behavior/Sub-Phase #1/Custom Discrete PD (Attitude) ==
  ez : Inport
  Sum3 : Sum
  kd_tr : Gain  Gain=Kd_tr
  kp_tr : Gain  Gain=Kp_tr
  "x_dot -> x1" : Subsystem
  Tz : Outport  VectorParamsAs1DForOutWhenUnconnected=off
  wires:
  kd_tr/1 -> Sum3/1
  Sum3/1 -> Tz/1
  kp_tr/1 -> Sum3/2
  "x_dot -> x1"/1(dy(t)/dt) -> kd_tr/1
  ez/1 -> "x_dot -> x1"/1(y(t)), kp_tr/1

== system MPC_Validation_2/Phase #3: Experiment/Change RED Behavior/Sub-Phase #1/Custom Discrete PD (X-Position) ==
  ex : Inport
  Sum3 : Sum
  kd_xr : Gain  Gain=Kd_xr
  kp_xr : Gain  Gain=Kp_xr
  "x_dot -> x1" : Subsystem
  Fx : Outport  VectorParamsAs1DForOutWhenUnconnected=off
  wires:
  kd_xr/1 -> Sum3/1
  ex/1 -> "x_dot -> x1"/1(y(t)), kp_xr/1
  kp_xr/1 -> Sum3/2
  "x_dot -> x1"/1(dy(t)/dt) -> kd_xr/1
  Sum3/1 -> Fx/1

== system MPC_Validation_2/Phase #3: Experiment/Change RED Behavior/Sub-Phase #1/Custom Discrete PD (Y-Position) ==
  ey : Inport
  Sum3 : Sum
  kd_yr : Gain  Gain=Kd_yr
  kp_yr : Gain  Gain=Kp_yr
  "x_dot -> x1" : Subsystem
  Fy : Outport  VectorParamsAs1DForOutWhenUnconnected=off
  wires:
  kd_yr/1 -> Sum3/1
  Sum3/1 -> Fy/1
  kp_yr/1 -> Sum3/2
  "x_dot -> x1"/1(dy(t)/dt) -> kd_yr/1
  ey/1 -> "x_dot -> x1"/1(y(t)), kp_yr/1

== system MPC_Validation_2/Phase #3: Experiment/Change RED Behavior/Sub-Phase #1/Hough Control ==
  Ref : Inport
  Act : Inport  Port=2
  MATLAB Function2 : MATLAB Function  TreatAsAtomicUnit=on
  MATLAB Function3 : MATLAB Function  TreatAsAtomicUnit=on
  MATLAB Function4 : MATLAB Function  TreatAsAtomicUnit=on
  Subtract2 : Sum  Inputs=+-
  Err : Outport  VectorParamsAs1DForOutWhenUnconnected=off
  wires:
  MATLAB Function4/1(e_out) -> Err/1
  MATLAB Function2/1(Oy) -> MATLAB Function4/1(Oy)
  Subtract2/1 -> MATLAB Function4/2(e_in)
  MATLAB Function2/2(Ox) -> Subtract2/1
  Act/1 -> MATLAB Function3/1(z)
  Ref/1 -> MATLAB Function2/1(z)
  MATLAB Function3/1(Ox) -> Subtract2/2

== system MPC_Validation_2/Phase #3: Experiment/Change RED Behavior/Sub-Phase #1/RED ==
  note: ARM Control Law - RED
  note: When the ARM is not in use, send zeros.
  Action Port : ActionPort  ActionPortLabel=else
  Constant7 : Constant  Value=0
  RED_Fx1 : DataStoreWrite  DataStoreName=RED_Tz_Shoulder
  RED_Fy1 : DataStoreWrite  DataStoreName=RED_Tz_Elbow
  RED_Tz1 : DataStoreWrite  DataStoreName=RED_Tz_Wrist
  wires:
  Constant7/1 -> RED_Fx1/1, RED_Fy1/1, RED_Tz1/1

== system MPC_Validation_2/Phase #3: Experiment/Change RED Behavior/Sub-Phase #1/RED+ARM ==
  note: ARM Control Law - RED
  note: This section is reserved for any control law for the robotic manipulator.
  Action Port : ActionPort  ActionPortLabel=if(u1 == 4 | u1 == 5 | u1 == 10 | u1 == 11)
  Constant7 : Constant  Value=0
  Constant8 : Constant  Value=pi/2
  Constant9 : Constant  Value=pi/2
  Custom Discrete PD (X-Position)1 : Subsystem
  Custom Discrete PD (Y-Position)1 : Subsystem
  Custom Discrete PD (Y-Position)2 : Subsystem
  RED_Fx1 : DataStoreWrite  DataStoreName=RED_Tz_Shoulder
  RED_Fy1 : DataStoreWrite  DataStoreName=RED_Tz_Elbow
  RED_Px1 : DataStoreRead  DataStoreName=RED_Rz_Shoulder
  RED_Px2 : DataStoreRead  DataStoreName=RED_Rz_Elbow
  RED_Rz1 : DataStoreRead  DataStoreName=RED_Rz_Wrist
  RED_Tz1 : DataStoreWrite  DataStoreName=RED_Tz_Wrist
  Saturation : Saturate  UpperLimit=Tz_lim_sharm  LowerLimit=-Tz_lim_sharm
  Saturation1 : Saturate  UpperLimit=Tz_lim_elarm  LowerLimit=-Tz_lim_elarm
  Saturation3 : Saturate  UpperLimit=Tz_lim_wrarm  LowerLimit=-Tz_lim_wrarm
  Subtract2 : Sum  Inputs=+-
  Subtract3 : Sum  Inputs=+-
  Subtract4 : Sum  Inputs=+-
  wires:
  Saturation3/1 -> RED_Tz1/1
  Custom Discrete PD (Y-Position)1/1(Fy) -> Saturation1/1
  Saturation1/1 -> RED_Fy1/1
  Constant9/1 -> Subtract3/1
  Subtract3/1 -> Custom Discrete PD (Y-Position)1/1(ey)
  RED_Px2/1 -> Subtract3/2
  RED_Rz1/1 -> Subtract4/2
  Custom Discrete PD (X-Position)1/1(Fx) -> Saturation/1
  Constant8/1 -> Subtract2/1
  Custom Discrete PD (Y-Position)2/1(Fy) -> Saturation3/1
  Constant7/1 -> Subtract4/1
  Subtract4/1 -> Custom Discrete PD (Y-Position)2/1(ey)
  Saturation/1 -> RED_Fx1/1
  RED_Px1/1 -> Subtract2/2
  Subtract2/1 -> Custom Discrete PD (X-Position)1/1(ex)

== system MPC_Validation_2/Phase #3: Experiment/Change RED Behavior/Sub-Phase #2 /RED ==
  note: ARM Control Law - RED
  note: When the ARM is not in use, send zeros.
  Action Port : ActionPort  ActionPortLabel=else
  Constant7 : Constant  Value=0
  RED_Fx1 : DataStoreWrite  DataStoreName=RED_Tz_Shoulder
  RED_Fy1 : DataStoreWrite  DataStoreName=RED_Tz_Elbow
  RED_Tz1 : DataStoreWrite  DataStoreName=RED_Tz_Wrist
  wires:
  Constant7/1 -> RED_Fx1/1, RED_Fy1/1, RED_Tz1/1

== system MPC_Validation_2/Phase #3: Experiment/Change RED Behavior/Sub-Phase #2 /RED+ARM ==
  note: ARM Control Law - RED
  note: This section is reserved for any control law for the robotic manipulator.
  Action Port : ActionPort  ActionPortLabel=if(u1 == 4 | u1 == 5 | u1 == 10 | u1 == 11)
  Constant7 : Constant  Value=0
  Constant8 : Constant  Value=pi/2
  Constant9 : Constant  Value=pi/2
  Custom Discrete PD (X-Position)1 : Subsystem
  Custom Discrete PD (Y-Position)1 : Subsystem
  Custom Discrete PD (Y-Position)2 : Subsystem
  RED_Fx1 : DataStoreWrite  DataStoreName=RED_Tz_Shoulder
  RED_Fy1 : DataStoreWrite  DataStoreName=RED_Tz_Elbow
  RED_Px1 : DataStoreRead  DataStoreName=RED_Rz_Shoulder
  RED_Px2 : DataStoreRead  DataStoreName=RED_Rz_Elbow
  RED_Rz1 : DataStoreRead  DataStoreName=RED_Rz_Wrist
  RED_Tz1 : DataStoreWrite  DataStoreName=RED_Tz_Wrist
  Saturation : Saturate  UpperLimit=Tz_lim_sharm  LowerLimit=-Tz_lim_sharm
  Saturation1 : Saturate  UpperLimit=Tz_lim_elarm  LowerLimit=-Tz_lim_elarm
  Saturation3 : Saturate  UpperLimit=Tz_lim_wrarm  LowerLimit=-Tz_lim_wrarm
  Subtract2 : Sum  Inputs=+-
  Subtract3 : Sum  Inputs=+-
  Subtract4 : Sum  Inputs=+-
  wires:
  Saturation3/1 -> RED_Tz1/1
  Custom Discrete PD (Y-Position)1/1(Fy) -> Saturation1/1
  Saturation1/1 -> RED_Fy1/1
  Constant9/1 -> Subtract3/1
  Subtract3/1 -> Custom Discrete PD (Y-Position)1/1(ey)
  RED_Px2/1 -> Subtract3/2
  RED_Rz1/1 -> Subtract4/2
  Custom Discrete PD (X-Position)1/1(Fx) -> Saturation/1
  Constant8/1 -> Subtract2/1
  Custom Discrete PD (Y-Position)2/1(Fy) -> Saturation3/1
  Constant7/1 -> Subtract4/1
  Subtract4/1 -> Custom Discrete PD (Y-Position)2/1(ey)
  Saturation/1 -> RED_Fx1/1
  RED_Px1/1 -> Subtract2/2
  Subtract2/1 -> Custom Discrete PD (X-Position)1/1(ex)

== system MPC_Validation_2/Phase #3: Experiment/Change RED Behavior/Sub-Phase #3 /RED ==
  note: ARM Control Law - RED
  note: When the ARM is not in use, send zeros.
  Action Port : ActionPort  ActionPortLabel=else
  Constant7 : Constant  Value=0
  RED_Fx1 : DataStoreWrite  DataStoreName=RED_Tz_Shoulder
  RED_Fy1 : DataStoreWrite  DataStoreName=RED_Tz_Elbow
  RED_Tz1 : DataStoreWrite  DataStoreName=RED_Tz_Wrist
  wires:
  Constant7/1 -> RED_Fx1/1, RED_Fy1/1, RED_Tz1/1
